simulink model "TrajectoryFollower"  (R2022a)
settings: Solver=FixedStepAuto  StartTime=0.0  StopTime=10.0  RelTol=1e-3
libraries: robotcorelib x1, robotalgslib x1
settings Model: Creator=The MathWorks, Inc.  LastModifiedBy=The MathWorks, Inc.
settings SolverCC: AlgebraicLoopSolver=TrustRegion  MaxZcPerStep=1
settings DebuggingCC: UnconnectedInputMsg=warning  UnconnectedOutputMsg=warning  UnconnectedLineMsg=warning  SFMachineParentedDataDiag=warning
settings ModelReferenceCC: ModelReferenceNumInstancesAllowed=Single
settings RTWCC: DLArmComputeVersion=19.05

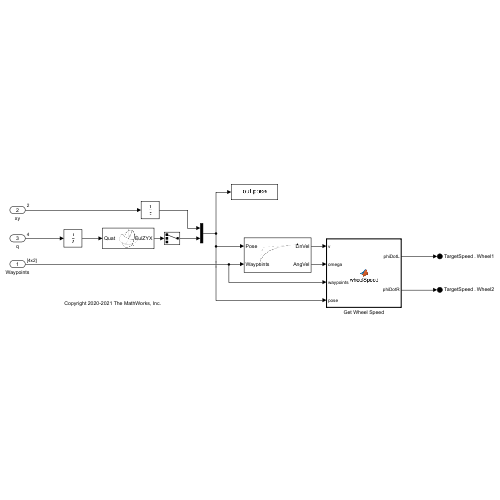
[thumbnail: Simulink's stored preview of the top-level diagram]
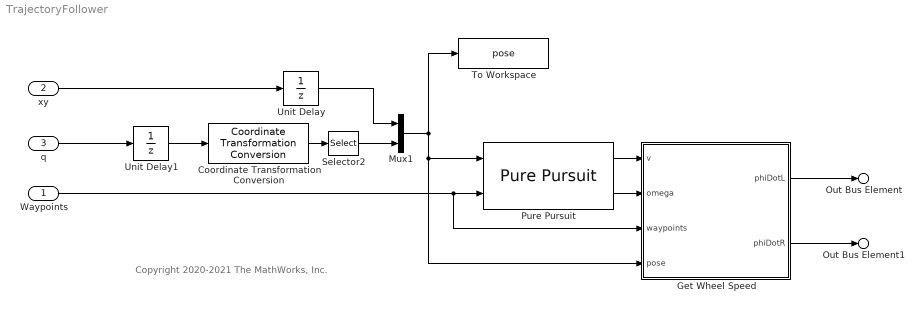
== system TrajectoryFollower ==
  note: Copyright 2020-2021 The MathWorks, Inc.
  Waypoints : Inport  PortDimensions=[4,2]
  xy : Inport  Port=2  PortDimensions=2  SampleTime=0.001
  q : Inport  Port=3  PortDimensions=4  SampleTime=0.001
  Coordinate Transformation Conversion : robotcorelib/Coordinate Transformation Conversion  InputRepresentation=Quaternion  InputEulerSequence=ZYX  ShowTrVecInputPort=on  OutputRepresentation=Euler Angles  OutputEulerSequence=ZYX  ShowTrVecOutputPort=on  SimulateUsing=Code generation
      settings: SourceProductBaseCode=RO,NV,RR,UV
  Get Wheel Speed : MATLAB Function  TreatAsAtomicUnit=on
  Mux1 : Mux  Inputs=2
  Pure Pursuit : robotalgslib/Pure Pursuit  DesiredLinearVelocity=0.5  MaxAngularVelocity=pi/2  LookaheadDistance=0.5  TargetDirPort=off  SimulateUsing=Code generation
  Selector2 : Selector  InputPortWidth=3  IndexOptions=Index vector (dialog)  Indices=1  OutputSizes=1
  To Workspace : ToWorkspace  VariableName=pose  SaveFormat=Timeseries  SampleTime=-1
  Unit Delay : UnitDelay  InitialCondition=[0 0]  SampleTime=-1  HasFrameUpgradeWarning=on
  Unit Delay1 : UnitDelay  InitialCondition=[1 0 0 0]  SampleTime=-1  HasFrameUpgradeWarning=on
  Out Bus Element : Outport  PortName=TargetSpeed  Element=Wheel1
  Out Bus Element1 : Outport  PortName=TargetSpeed  Element=Wheel2
  wires:
  Get Wheel Speed/1(phiDotL) -> Out Bus Element/1
  Coordinate Transformation Conversion/1 -> Selector2/1
  Pure Pursuit/2 -> Get Wheel Speed/2(omega)
  Pure Pursuit/1 -> Get Wheel Speed/1(v)
  Get Wheel Speed/2(phiDotR) -> Out Bus Element1/1
  Unit Delay1/1 -> Coordinate Transformation Conversion/1
  xy/1 -> Unit Delay/1
  Mux1/1 -> Get Wheel Speed/4(pose), Pure Pursuit/1, To Workspace/1
  Selector2/1 -> Mux1/2
  Unit Delay/1 -> Mux1/1
  q/1 -> Unit Delay1/1
  Waypoints/1 -> Get Wheel Speed/3(waypoints), Pure Pursuit/2

== matlab function TrajectoryFollower/Get Wheel Speed ==
  data: v input; omega input; waypoints input; pose input; phiDotL output; phiDotR output
function [phiDotL, phiDotR] = wheelSpeed(v, omega, waypoints, pose)

% Path constants
stopThreshold = 0.1;
slowThreshold = 0.2;

% Robot constants 
trackWidth = 0.3;
wheelRadius = 0.1;

% Slow the robot down when it's near the threshold
distanceToEndpoint = norm(waypoints(end, :) - pose(1:2)');
if (distanceToEndpoint < slowThreshold)
    v = distanceToEndpoint/slowThreshold*v;
    
    % Stop the robot if it's inside the target threshold
    if distanceToEndpoint < stopThreshold
        v = 0;
    end
end

% Convert velocity and heading angular velocity to wheel speeds
phiDotL = (v - trackWidth/2*omega)/wheelRadius;
phiDotR = (v + trackWidth/2*omega)/wheelRadius;

end
